simulink library "Electric_Heating"  (R2016b)
settings: Solver=ode45  StartTime=0.0  StopTime=10.0  RelTol=1e-3  EnableMultiTasking=on
undefined symbols (not defined in the file): nodes
settings Model: Creator=lena.frank  LastModifiedBy=drhf
settings DataIOCC: LimitDataPoints=on  SaveFormat=Array  SignalLoggingSaveFormat=ModelDataLogs
settings OptimizationCC: ExpressionDepthLimit=2147483647  LifeSpan=inf
settings DebuggingCC: UnderspecifiedInitializationDetection=Classic  MergeDetectMultiDrivingBlocksExec=none  SolverPrmCheckMsg=warning  FcnCallInpInsideContextMsg=warning  StateNameClashWarn=warning  SFUnexpectedBacktrackingDiag=warning  SFNoUnconditionalDefaultTransitionDiag=warning  SFExecutionAtInitializationDiag=none
settings HardwareCC: ProdBitPerPointer=32  ProdBitPerSizeT=32  ProdBitPerPtrDiffT=32  ProdLargestAtomicFloat=None  ProdIntDivRoundTo=Undefined  ProdEndianess=Unspecified  ProdWordSize=32  ProdHWDeviceType=32-bit Generic
settings ModelReferenceCC: PropagateSignalLabelsOutOfModel=off
settings GRTTargetCC: TargetLangStandard=C89/C90 (ANSI)  GeneratePreprocessorConditionals=Disable all  CombineOutputUpdateFcns=off  GRTInterface=on
settings ConfigComp: CovMetricSettings=dw  CovHtmlReporting=on  CovSaveCumulativeToWorkspaceVar=on  CovSaveSingleToWorkspaceVar=on  CovExternalEMLEnable=off

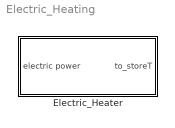
== system Electric_Heating ==
  Electric_Heater : Subsystem  mask(electric heating){hin=0, hout=0.4, nodes=nodes}
      mask prompts: hin "relative height start heating zone"; hout "relative height end heating zone"; nodes "Number of nodes (do not change here)"
      mask help: The block is an electric backup heating for the storage. Give inlet- and outlet-height as a relative position from 0 (= bottom) to 1 (= top).
      mask init:
      | hin = min(1, max(0, hin));
      | hout = min(1, max(0, hout));
      | 
      | if hin < hout
      |     inlet = max(ceil(hin*nodes),1);    % start node of heated zone
      |     outlet = max(ceil(hout*nodes),1);  % end node of heated zone
      | else
      |     outlet = max(ceil(hin*nodes),1);   % end node of heated zone
      |     inlet = max(ceil(hout*nodes),1);   % start node of heated zone
      | end
      | 
      | Q = zeros(nodes,1);                    % initilize power vector
      | if inlet < outlet
      |     Q(inlet:outlet) = ones(outlet-inlet+1,1); % set heated zone to One
      | else
      |     Q(outlet:inlet) = ones(inlet-outlet+1,1); % set heated zone to One
      | end
      | Q = Q./sum(Q);                         % sum over all elements must be one
      mask Help: web(fullfile(path_carnot('help'),'Electric_Heating.html'),'-helpbrowser')
      mask Display: disp('Electric\n\nHeater')

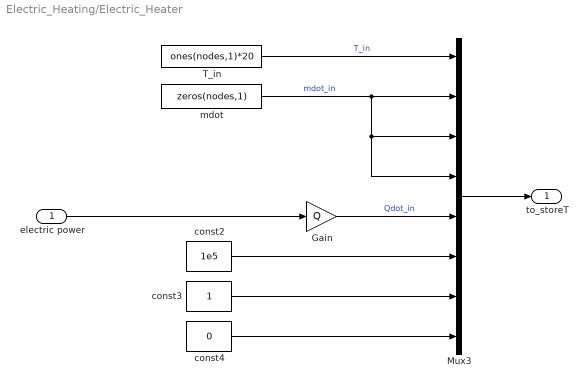
== system Electric_Heating/Electric_Heater ==
  electric power : Inport
  Gain : Gain  Gain=Q
  Mux3 : Mux  Inputs=8
  T_in : Constant  Value=ones(nodes,1)*20
  const2 : Constant  Value=1e5
  const3 : Constant
  const4 : Constant  Value=0
  mdot : Constant  Value=zeros(nodes,1)
  to_storeT : Outport
  wires:
  Gain/1 -> Mux3/5  "Qdot_in"
  const4/1 -> Mux3/8
  electric power/1 -> Gain/1
  T_in/1 -> Mux3/1  "T_in"
  Mux3/1 -> to_storeT/1
  mdot/1 -> Mux3/4, Mux3/3, Mux3/2  "mdot_in"
  const2/1 -> Mux3/6
  const3/1 -> Mux3/7
